simulink model "test_compressible_line"  (R2013a)
settings: Solver=ode15s  StartTime=0.0  StopTime=0.05  RelTol=1e-5
undefined symbols (not defined in the file): L
libraries: usask_hyd_lib x4, fl_lib x3, nesl_utility x2
settings Model: Creator=tkw954  LastModifiedBy=tkw954

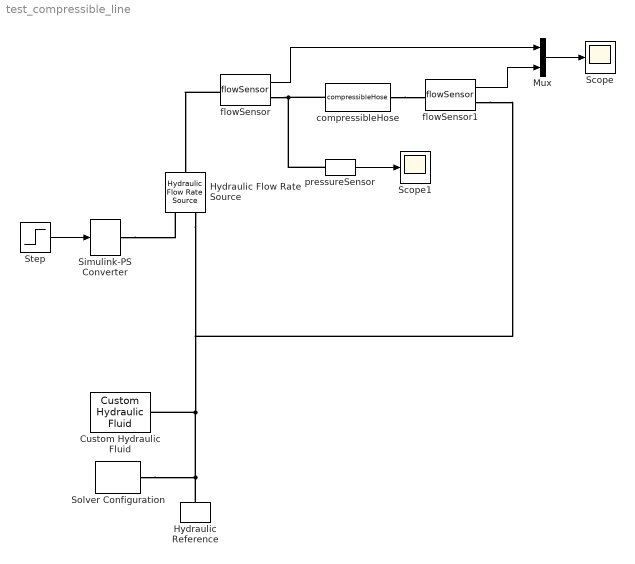
== system test_compressible_line ==
  Custom Hydraulic Fluid : fl_lib/Hydraulic/Hydraulic Utilities/Custom Hydraulic Fluid  density=850 kg/m^3  viscosity_kin=18e-6 m^2/s  bulk=0.8e9 Pa  alpha=0.005  LocalVarLogging=[]
  Hydraulic Flow Rate Source : fl_lib/Hydraulic/Hydraulic Sources/Hydraulic Flow Rate Source  q_Log=off  p_Log=off  LocalVarNames=|q|p  LocalVarDescs=|q|p  LocalVarLogging=[0 0]
  Hydraulic Reference : fl_lib/Hydraulic/Hydraulic Elements/Hydraulic Reference  q_Log=off  LocalVarNames=|q  LocalVarDescs=|q  LocalVarLogging=0
  Mux : Mux  Inputs=2
  Scope : Scope
  Scope1 : Scope
  Simulink-PS Converter : nesl_utility/Simulink-PS Converter  PhysicalDomain=network_engine_domain  SubClassName=ps_input  LeftPortType=input  RightPortType=output  PseudoPeriodic=off  Frequencies=[]  NoiseDistribution=none  NoiseParameters=[]  Unit=1  AffineConversion=off  InputFiltering=off  SimscapeFilterOrder=1  InputFilterTimeConstant=0.001  UdotUserProvided=1
  Solver Configuration : nesl_utility/Solver Configuration  PhysicalDomain=network_engine_domain  SubClassName=solver  LeftPortType=input  RightPortType=generic  Accelerate=off  Tones=[]  Harmonics=[]  SimulateNoise=off  Profile=off  UseLocalSampling=off  EnableSwitchedLinearOptims=on  FrequencyDomain=off  UseCCode=off  UseNewInitialization=off  DoDC=off  ResidualTolerance=1e-09  UseLocalSolver=off  LocalSolverChoice=NE_BACKWARD_EULER_ADVANCER  LocalSolverSampleTime=0.001  DoFixedCost=off  MaxNonlinIter=3  MaxModeIter=2  LinearAlgebra=Sparse  DelaysMemoryBudget=1024
  Step : Step  Time=1e-2  After=100/60000  SampleTime=0
  compressibleHose : usask_hyd_lib/compressibleHose  d=12e-3  L=2  dd_dP=1.2e-12  P0=0  e=0
  flowSensor : usask_hyd_lib/flowSensor  unitNum=L/min
  flowSensor1 : usask_hyd_lib/flowSensor  unitNum=L/min
  pressureSensor : usask_hyd_lib/pressureSensor  unitNum=kPa
  wires:
  Step/1 -> Simulink-PS Converter/1
  flowSensor/1 -> Mux/1
  flowSensor1/1 -> Mux/2
  Mux/1 -> Scope/1
  pressureSensor/1 -> Scope1/1
  connections:
  Hydraulic Reference/LConn1 -- Solver Configuration/RConn1 -- flowSensor1/RConn1 -- Hydraulic Flow Rate Source/RConn2 -- Custom Hydraulic Fluid/RConn1
  Simulink-PS Converter/RConn1 -- Hydraulic Flow Rate Source/RConn1
  flowSensor/RConn1 -- compressibleHose/LConn1 -- pressureSensor/LConn1
  flowSensor/LConn1 -- Hydraulic Flow Rate Source/LConn1
  compressibleHose/RConn1 -- flowSensor1/LConn1
